simulink model "CF016A_GmVehSpdArbn"  (R2013b)
settings: Solver=FixedStepDiscrete  SolverMode=SingleTasking  StartTime=0.0  StopTime=1  FixedStep=0.002  RelTol=1e-3
undefined symbols (not defined in the file): DIAGCSTRTUPDLY_CNT_U32, NODEBSTEP_CNT_U16, NtcNr1, NtcSts1, VEHSPDMAX_KPH_F32
libraries: simulink x8, NxtrMax x7, NxtrMin x3, NxtrLim x3
(part 2 of 5)

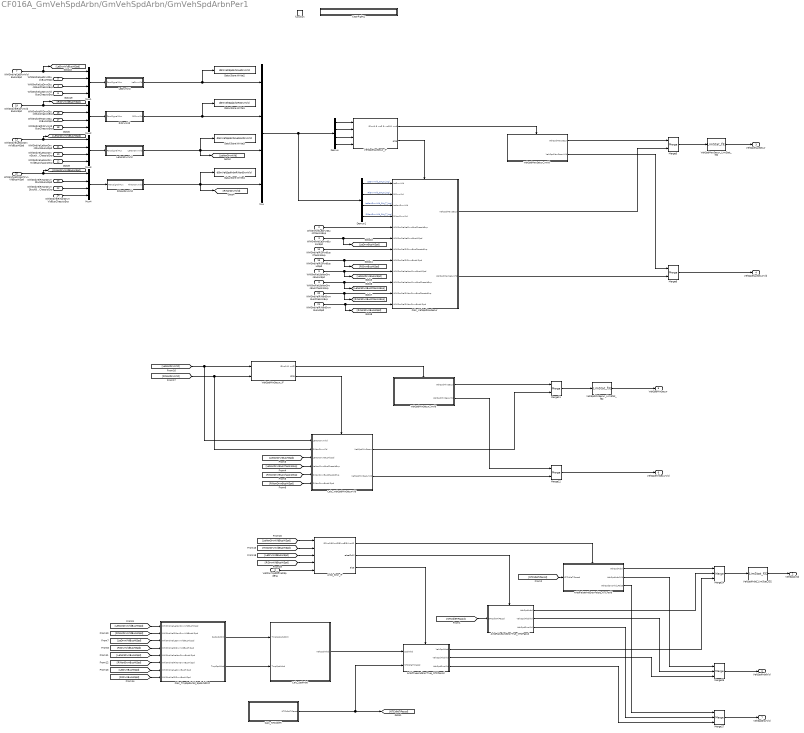
== system CF016A_GmVehSpdArbn/GmVehSpdArbn/GmVehSpdArbnPer1 ==
  VehPwrModDftVehSpdEna : Inport  RequirementInfo="{'linktype_rmi_doors' '0000c6e6 (/GM T1XX/SubSystem Specifications/Customer Functions/CF016A GM Vehicle Speed Arbitration)' '#201' 'true' 'REQ:  201' '' ; 'linktype_rmi_doors' '0000c6e6 (/GM T1XX/SubSystem Specifications/Customer Functions/CF016A GM Vehicle Speed Arbitration)' '#216' 'true' 'REQ:  216' '' ; 'linktype_rmi_doors' '0000c6e6 (/GM T1XX/SubSystem Specifications/Customer Functions/CF016A GM Vehicle Speed Arbitration)' '#55' 'true' 'REQ:  55' '' ; 'linktype_rmi_doors' '0000c6e6 (/GM T1XX/SubSystem Specifications/Customer Functions/CF016A GM Vehicle Speed Arbitration)' '#21' 'true' 'REQ:  21' '' } %GIDa_c4e3bc18_0570_4b3f_a567_ab326b125ca6"  OutDataTypeStr=boolean
  WhlGndVelLeDrvnBusChassisExp : Inport  RequirementInfo="{'linktype_rmi_doors' '0000c6e6 (/GM T1XX/SubSystem Specifications/Customer Functions/CF016A GM Vehicle Speed Arbitration)' '#191' 'true' 'REQ:  191' '' } %GIDa_ef8bad56_b133_4efc_80e4_91ff1fcc71c4"  Port=2
  WhlGndVelLeDrvnBusHiSpd : Inport  RequirementInfo="{'linktype_rmi_doors' '0000c6e6 (/GM T1XX/SubSystem Specifications/Customer Functions/CF016A GM Vehicle Speed Arbitration)' '#191' 'true' 'REQ:  191' '' } %GIDa_139f3ad9_9f11_4eb8_ab0a_dd581ed38c16"  Port=3  OutDataTypeStr=single
  WhlGndVelLeDrvnStuckBusChassisExp : Inport  RequirementInfo="{'linktype_rmi_doors' '0000c6e6 (/GM T1XX/SubSystem Specifications/Customer Functions/CF016A GM Vehicle Speed Arbitration)' '#134' 'true' 'REQ:  134' '' } %GIDa_c2bb7793_67d4_43d9_8d0a_b84d2c7b072b"  Port=4  OutDataTypeStr=boolean
  WhlGndVelLeDrvnStuckBusHiSpd : Inport  RequirementInfo="{'linktype_rmi_doors' '0000c6e6 (/GM T1XX/SubSystem Specifications/Customer Functions/CF016A GM Vehicle Speed Arbitration)' '#134' 'true' 'REQ:  134' '' } %GIDa_c2f775a0_a216_4248_84ff_240bf61a6a65"  Port=5  OutDataTypeStr=boolean
  WhlGndVelLeDrvnVldBusChassisExp : Inport  RequirementInfo="{'linktype_rmi_doors' '0000c6e6 (/GM T1XX/SubSystem Specifications/Customer Functions/CF016A GM Vehicle Speed Arbitration)' '#134' 'true' 'REQ:  134' '' } %GIDa_795613aa_d3d4_4fbe_b3d8_2164d5b0da85"  Port=6  OutDataTypeStr=boolean
  WhlGndVelLeDrvnVldBusHiSpd : Inport  RequirementInfo="{'linktype_rmi_doors' '0000c6e6 (/GM T1XX/SubSystem Specifications/Customer Functions/CF016A GM Vehicle Speed Arbitration)' '#134' 'true' 'REQ:  134' '' } %GIDa_19a58a62_ea8b_42ac_976c_f323a4e5fb4e"  Port=7  OutDataTypeStr=boolean
  WhlGndVelLeNonDrvnBusChassisExp : Inport  RequirementInfo="{'linktype_rmi_doors' '0000c6e6 (/GM T1XX/SubSystem Specifications/Customer Functions/CF016A GM Vehicle Speed Arbitration)' '#191' 'true' 'REQ:  191' '' } %GIDa_816f3292_2a80_407e_aff3_aeaf91f0e3dd"  Port=8  OutDataTypeStr=single
  WhlGndVelLeNonDrvnBusHiSpd : Inport  RequirementInfo="{'linktype_rmi_doors' '0000c6e6 (/GM T1XX/SubSystem Specifications/Customer Functions/CF016A GM Vehicle Speed Arbitration)' '#191' 'true' 'REQ:  191' '' } %GIDa_66072834_5e26_43f6_80a8_02e13e05472d"  Port=9  OutDataTypeStr=single
  WhlGndVelLeNonDrvnStuckBusChassisExp : Inport  RequirementInfo="{'linktype_rmi_doors' '0000c6e6 (/GM T1XX/SubSystem Specifications/Customer Functions/CF016A GM Vehicle Speed Arbitration)' '#164' 'true' 'REQ:  164' '' } %GIDa_721a9ccb_d43e_4602_b1ac_eff13d3c585f"  Port=10  OutDataTypeStr=boolean
  WhlGndVelLeNonDrvnStuckBusHiSpd : Inport  RequirementInfo="{'linktype_rmi_doors' '0000c6e6 (/GM T1XX/SubSystem Specifications/Customer Functions/CF016A GM Vehicle Speed Arbitration)' '#164' 'true' 'REQ:  164' '' } %GIDa_3e912ca7_7856_471d_9266_b6036fbfae10"  Port=11  OutDataTypeStr=boolean
  WhlGndVelLeNonDrvnVldBusChassisExp : Inport  RequirementInfo="{'linktype_rmi_doors' '0000c6e6 (/GM T1XX/SubSystem Specifications/Customer Functions/CF016A GM Vehicle Speed Arbitration)' '#164' 'true' 'REQ:  164' '' } %GIDa_c6bce6c8_b68d_4bb8_bf53_f5356151d1e8"  Port=12  OutDataTypeStr=boolean
  WhlGndVelLeNonDrvnVldBusHiSpd : Inport  RequirementInfo="{'linktype_rmi_doors' '0000c6e6 (/GM T1XX/SubSystem Specifications/Customer Functions/CF016A GM Vehicle Speed Arbitration)' '#164' 'true' 'REQ:  164' '' } %GIDa_c358ba99_35ee_4eda_aec4_59a7f9c2cd81"  Port=13  OutDataTypeStr=boolean
  WhlGndVelRiDrvnBusChassisExp : Inport  RequirementInfo="{'linktype_rmi_doors' '0000c6e6 (/GM T1XX/SubSystem Specifications/Customer Functions/CF016A GM Vehicle Speed Arbitration)' '#191' 'true' 'REQ:  191' '' } %GIDa_5439fa4c_592a_4772_9e24_8e09c86df0d9"  Port=14  OutDataTypeStr=single
  WhlGndVelRiDrvnBusHiSpd : Inport  RequirementInfo="{'linktype_rmi_doors' '0000c6e6 (/GM T1XX/SubSystem Specifications/Customer Functions/CF016A GM Vehicle Speed Arbitration)' '#191' 'true' 'REQ:  191' '' } %GIDa_86c7eb5f_4f31_4eb8_8830_e40c7608a3bf"  Port=15  OutDataTypeStr=single
  WhlGndVelRiDrvnStuckBusChassisExp : Inport  RequirementInfo="{'linktype_rmi_doors' '0000c6e6 (/GM T1XX/SubSystem Specifications/Customer Functions/CF016A GM Vehicle Speed Arbitration)' '#148' 'true' 'REQ:  148' '' } %GIDa_585d7967_0ef8_49d7_8f11_a16ff24051d9"  Port=16  OutDataTypeStr=boolean
  WhlGndVelRiDrvnStuckBusHiSpd : Inport  RequirementInfo="{'linktype_rmi_doors' '0000c6e6 (/GM T1XX/SubSystem Specifications/Customer Functions/CF016A GM Vehicle Speed Arbitration)' '#148' 'true' 'REQ:  148' '' } %GIDa_76749fa7_0454_416a_acff_281ae28f658b"  Port=17  OutDataTypeStr=boolean
  WhlGndVelRiDrvnVldBusChassisExp : Inport  RequirementInfo="{'linktype_rmi_doors' '0000c6e6 (/GM T1XX/SubSystem Specifications/Customer Functions/CF016A GM Vehicle Speed Arbitration)' '#148' 'true' 'REQ:  148' '' } %GIDa_926dc97e_3db9_4017_9435_0a4137e9631c"  Port=18  OutDataTypeStr=boolean
  WhlGndVelRiDrvnVldBusHiSpd : Inport  RequirementInfo="{'linktype_rmi_doors' '0000c6e6 (/GM T1XX/SubSystem Specifications/Customer Functions/CF016A GM Vehicle Speed Arbitration)' '#148' 'true' 'REQ:  148' '' } %GIDa_5fab8672_ee1b_46d3_b7a0_1f2522ac3128"  Port=19  OutDataTypeStr=boolean
  WhlGndVelRiNonDrvnBusChassisExp : Inport  RequirementInfo="{'linktype_rmi_doors' '0000c6e6 (/GM T1XX/SubSystem Specifications/Customer Functions/CF016A GM Vehicle Speed Arbitration)' '#191' 'true' 'REQ:  191' '' } %GIDa_0d94133d_0a6e_49b6_947e_7364e274fe67"  Port=20  OutDataTypeStr=single
  WhlGndVelRiNonDrvnBusHiSpd : Inport  RequirementInfo="{'linktype_rmi_doors' '0000c6e6 (/GM T1XX/SubSystem Specifications/Customer Functions/CF016A GM Vehicle Speed Arbitration)' '#191' 'true' 'REQ:  191' '' } %GIDa_38490758_a269_42a5_8fec_e940c94565d1"  Port=21  OutDataTypeStr=single
  WhlGndVelRiNonDrvnStuckBusChassisExp : Inport  RequirementInfo="{'linktype_rmi_doors' '0000c6e6 (/GM T1XX/SubSystem Specifications/Customer Functions/CF016A GM Vehicle Speed Arbitration)' '#165' 'true' 'REQ:  165' '' } %GIDa_e0cb1563_d840_4dd2_a90a_2d810a7a7354"  Port=22  OutDataTypeStr=boolean
  WhlGndVelRiNonDrvnStuckBusHiSpd : Inport  RequirementInfo="{'linktype_rmi_doors' '0000c6e6 (/GM T1XX/SubSystem Specifications/Customer Functions/CF016A GM Vehicle Speed Arbitration)' '#165' 'true' 'REQ:  165' '' } %GIDa_e31240b4_81cc_4ab0_98ca_8ec14bb44c74"  Port=23  OutDataTypeStr=boolean
  WhlGndVelRiNonDrvnVldBusChassisExp : Inport  RequirementInfo="{'linktype_rmi_doors' '0000c6e6 (/GM T1XX/SubSystem Specifications/Customer Functions/CF016A GM Vehicle Speed Arbitration)' '#165' 'true' 'REQ:  165' '' } %GIDa_7a5865c5_6788_4082_bc3e_71db9840dce9"  Port=24  OutDataTypeStr=boolean
  WhlGndVelRiNonDrvnVldBusHiSpd : Inport  RequirementInfo="{'linktype_rmi_doors' '0000c6e6 (/GM T1XX/SubSystem Specifications/Customer Functions/CF016A GM Vehicle Speed Arbitration)' '#165' 'true' 'REQ:  165' '' } %GIDa_97efc4a3_badf_4f9c_a1b1_7d9397b8ff86"  Port=25  OutDataTypeStr=boolean
  function : TriggerPort  TriggerType=function-call
  ArbdFalseAndSnsrFalse_NTCFaild : Subsystem  RequirementInfo="{'linktype_rmi_doors' '0000c6e6 (/GM T1XX/SubSystem Specifications/Customer Functions/CF016A GM Vehicle Speed Arbitration)' '#201' 'true' 'REQ:  201' '' ; 'linktype_rmi_doors' '0000c6e6 (/GM T1XX/SubSystem Specifications/Customer Functions/CF016A GM Vehicle Speed Arbitration)' '#216' 'true' 'REQ:  216' '' ; 'linktype_rmi_doors' '0000c6e6 (/GM T1XX/SubSystem Specifications/Customer Functions/CF016A GM Vehicle Speed Arbitration)' '#55' 'true' 'REQ:  55' '' } %GIDa_a2946cc7_76d5_475e_a7d4_3e59e6c0f436"  TreatAsAtomicUnit=on
  ArbdFalseAndSnsrTrue_NTCPassd : Subsystem  RequirementInfo="{'linktype_rmi_doors' '0000c6e6 (/GM T1XX/SubSystem Specifications/Customer Functions/CF016A GM Vehicle Speed Arbitration)' '#201' 'true' 'REQ:  201' '' ; 'linktype_rmi_doors' '0000c6e6 (/GM T1XX/SubSystem Specifications/Customer Functions/CF016A GM Vehicle Speed Arbitration)' '#216' 'true' 'REQ:  216' '' ; 'linktype_rmi_doors' '0000c6e6 (/GM T1XX/SubSystem Specifications/Customer Functions/CF016A GM Vehicle Speed Arbitration)' '#55' 'true' 'REQ:  55' '' ; 'linktype_rmi_doors' '0000c6e6 (/GM T1XX/SubSystem Specifications/Customer Functions/CF016A GM Vehicle Speed Arbitration)' '#21' 'true' 'REQ:  21' '' } %GIDa_24968ccd_650a_4f02_a76c_60fb17be485c"  TreatAsAtomicUnit=on
  ArbdTrueAndSnsrTrue_NTCPassd : Subsystem  RequirementInfo="{'linktype_rmi_doors' '0000c6e6 (/GM T1XX/SubSystem Specifications/Customer Functions/CF016A GM Vehicle Speed Arbitration)' '#201' 'true' 'REQ:  201' '' ; 'linktype_rmi_doors' '0000c6e6 (/GM T1XX/SubSystem Specifications/Customer Functions/CF016A GM Vehicle Speed Arbitration)' '#216' 'true' 'REQ:  216' '' ; 'linktype_rmi_doors' '0000c6e6 (/GM T1XX/SubSystem Specifications/Customer Functions/CF016A GM Vehicle Speed Arbitration)' '#55' 'true' 'REQ:  55' '' } %GIDa_a93f8941_36e9_423e_8493_7bbaddef002d"  TreatAsAtomicUnit=on
  Arbd_Snsr_IF : If  RequirementInfo="{'linktype_rmi_doors' '0000c6e6 (/GM T1XX/SubSystem Specifications/Customer Functions/CF016A GM Vehicle Speed Arbitration)' '#201' 'true' 'REQ:  201' '' ; 'linktype_rmi_doors' '0000c6e6 (/GM T1XX/SubSystem Specifications/Customer Functions/CF016A GM Vehicle Speed Arbitration)' '#216' 'true' 'REQ:  216' '' ; 'linktype_rmi_doors' '0000c6e6 (/GM T1XX/SubSystem Specifications/Customer Functions/CF016A GM Vehicle Speed Arbitration)' '#55' 'true' 'REQ:  55' '' ; 'linktype_rmi_doors' '0000c6e6 (/GM T1XX/SubSystem Specifications/Customer Functions/CF016A GM Vehicle Speed Arbitration)' '#21' 'true' 'REQ:  21' '' } %GIDa_cd7d7c1a_47a2_4b6f_81bf_446ff4509ba4"  NumInputs=5  IfExpression=(~u1)&(~u2)&(~u3)&(~u4)  ElseIfExpressions=u5
      settings: AttributesFormatString=|
      | IF: %<IfExpression>
      | ELSE IF: %<ElseIfExpressions>
  Calc_NTCIdleTi : Subsystem  RequirementInfo="{'linktype_rmi_doors' '0000c6e6 (/GM T1XX/SubSystem Specifications/Customer Functions/CF016A GM Vehicle Speed Arbitration)' '#223' 'true' 'REQ:  223' '' } %GIDa_b1c70a04_ae11_4796_80c0_e305c1af5713"
  Calc_SpdArbd : Subsystem  RequirementInfo="{'linktype_rmi_doors' '0000c6e6 (/GM T1XX/SubSystem Specifications/Customer Functions/CF016A GM Vehicle Speed Arbitration)' '#197' 'true' 'REQ:  197' '' } %GIDa_16311984_c18c_4fe4_ad8c_ca1138d95f11"
  Calc_TmpSpdArbd_SpdArbdCnt : Subsystem  RequirementInfo="{'linktype_rmi_doors' '0000c6e6 (/GM T1XX/SubSystem Specifications/Customer Functions/CF016A GM Vehicle Speed Arbitration)' '#197' 'true' 'REQ:  197' '' } %GIDa_bc6bf8a9_5351_4ff1_8876_c778375d82ed"
  Calc_VehSpdMaxSecur : Subsystem  RequirementInfo="{'linktype_rmi_doors' '0000c6e6 (/GM T1XX/SubSystem Specifications/Customer Functions/CF016A GM Vehicle Speed Arbitration)' '#42' 'true' 'REQ:  42' '' } %GIDa_18b5dd71_8b65_4e5b_b3d7_592b4660d087"  TreatAsAtomicUnit=on
  Calc_VehSpdMinSecurVld : Subsystem  RequirementInfo="{'linktype_rmi_doors' '0000c6e6 (/GM T1XX/SubSystem Specifications/Customer Functions/CF016A GM Vehicle Speed Arbitration)' '#200' 'true' 'REQ:  200' '' } %GIDa_87f42618_bdcc_4508_97d2_5a3f6cb92617"  TreatAsAtomicUnit=on
  CopyRight2 : Subsystem  Description=|  mask(Copyright Information){none=on}
      | Copyright info block.                                               
      |                                                                     
      | Place copyright information at the top of every subsystem in design.
      mask prompts: none "No parameters"
      mask help: Place copyright information at the top of every subsystem in design.
      mask Display:
      | NxtrConf = 'Nexteer Confidential';
      | 
      | sys = bdroot; %handle for the current model ("system")
      | first = get_param(sys,'Created');
      | if(isempty(first))
      |     first = datestr(now,'yyyy');
      | else
      |     first = first(end-3:end);  %year is last four digits
      | end
      | 
      | last = get_param(sys,'LastModifiedDate');
      | if isempty(last)
      |     last = datestr(now,'yyyy');
      | else
      |     last = last(end-3:end);
      | end
      | 
      | if strcmp(first,last)
      |     fprintf('%s -- Copyright %s Nexteer',NxtrConf,first)
      | else
      |     fprintf('%s -- %s%s- %s Nexteer',NxtrConf,char(169),first,last)
      | end
  Data Store Write1 : DataStoreWrite  RequirementInfo="{'linktype_rmi_doors' '0000c6e6 (/GM T1XX/SubSystem Specifications/Customer Functions/CF016A GM Vehicle Speed Arbitration)' '#148' 'true' 'REQ:  148' '' } %GIDa_65a22cee_f7c3_4e4f_9841_3f731132c91b"  DataStoreName=dGmVehSpdArbnRiDrvnVld
  Data Store Write2 : DataStoreWrite  RequirementInfo="{'linktype_rmi_doors' '0000c6e6 (/GM T1XX/SubSystem Specifications/Customer Functions/CF016A GM Vehicle Speed Arbitration)' '#134' 'true' 'REQ:  134' '' } %GIDa_6506a920_d21b_4a41_8912_67910f5698ca"  DataStoreName=dGmVehSpdArbnLeDrvnVld
  Data Store Write3 : DataStoreWrite  RequirementInfo="{'linktype_rmi_doors' '0000c6e6 (/GM T1XX/SubSystem Specifications/Customer Functions/CF016A GM Vehicle Speed Arbitration)' '#164' 'true' 'REQ:  164' '' } %GIDa_7caea8aa_01ba_480f_a0e3_d7874300fc26"  DataStoreName=dGmVehSpdArbnLeNonDrvnVld
  Data Store Write4 : DataStoreWrite  RequirementInfo="{'linktype_rmi_doors' '0000c6e6 (/GM T1XX/SubSystem Specifications/Customer Functions/CF016A GM Vehicle Speed Arbitration)' '#165' 'true' 'REQ:  165' '' } %GIDa_537405e5_2b08_46e6_bc5f_2c920737d5d3"  DataStoreName=dGmVehSpdArbnRiNonDrvnVld
  Demux : Demux  RequirementInfo="{'linktype_rmi_doors' '0000c6e6 (/GM T1XX/SubSystem Specifications/Customer Functions/CF016A GM Vehicle Speed Arbitration)' '#151' 'true' 'REQ:  151' '' } %GIDa_9996e851_1594_4344_ab35_741cd3cb2f5f"
  Demux1 : Demux
  LeDrvnVld : Subsystem  RequirementInfo="{'linktype_rmi_doors' '0000c6e6 (/GM T1XX/SubSystem Specifications/Customer Functions/CF016A GM Vehicle Speed Arbitration)' '#134' 'true' 'REQ:  134' '' } %GIDa_91d91c9c_e4ce_47bd_8edb_064a3de60f07"
  LeNonDrvnVld : Subsystem  RequirementInfo="{'linktype_rmi_doors' '0000c6e6 (/GM T1XX/SubSystem Specifications/Customer Functions/CF016A GM Vehicle Speed Arbitration)' '#164' 'true' 'REQ:  164' '' } %GIDa_738d4c5d_c85c_4fc7_a21b_b06397be08db"
  Merge11 : Merge  RequirementInfo="{'linktype_rmi_doors' '0000c6e6 (/GM T1XX/SubSystem Specifications/Customer Functions/CF016A GM Vehicle Speed Arbitration)' '#200' 'true' 'REQ:  200' '' } %GIDa_c6f44c10_058a_4ce8_bab9_d9e154170ef5"
  Merge12 : Merge  RequirementInfo="{'linktype_rmi_doors' '0000c6e6 (/GM T1XX/SubSystem Specifications/Customer Functions/CF016A GM Vehicle Speed Arbitration)' '#200' 'true' 'REQ:  200' '' } %GIDa_5ca221ae_a0a0_4349_801e_90a121427c6f"
  Merge24 : Merge  RequirementInfo="{'linktype_rmi_doors' '0000c6e6 (/GM T1XX/SubSystem Specifications/Customer Functions/CF016A GM Vehicle Speed Arbitration)' '#201' 'true' 'REQ:  201' '' ; 'linktype_rmi_doors' '0000c6e6 (/GM T1XX/SubSystem Specifications/Customer Functions/CF016A GM Vehicle Speed Arbitration)' '#216' 'true' 'REQ:  216' '' ; 'linktype_rmi_doors' '0000c6e6 (/GM T1XX/SubSystem Specifications/Customer Functions/CF016A GM Vehicle Speed Arbitration)' '#55' 'true' 'REQ:  55' '' } %GIDa_74dbaf74_bffd_42bd_8f7c_be8132b0f70d"  Inputs=3
  Merge25 : Merge  RequirementInfo="{'linktype_rmi_doors' '0000c6e6 (/GM T1XX/SubSystem Specifications/Customer Functions/CF016A GM Vehicle Speed Arbitration)' '#201' 'true' 'REQ:  201' '' ; 'linktype_rmi_doors' '0000c6e6 (/GM T1XX/SubSystem Specifications/Customer Functions/CF016A GM Vehicle Speed Arbitration)' '#216' 'true' 'REQ:  216' '' ; 'linktype_rmi_doors' '0000c6e6 (/GM T1XX/SubSystem Specifications/Customer Functions/CF016A GM Vehicle Speed Arbitration)' '#55' 'true' 'REQ:  55' '' } %GIDa_f96da6f3_b28c_497a_a08f_fa4ee1d04650"  Inputs=3
  Merge27 : Merge  RequirementInfo="{'linktype_rmi_doors' '0000c6e6 (/GM T1XX/SubSystem Specifications/Customer Functions/CF016A GM Vehicle Speed Arbitration)' '#201' 'true' 'REQ:  201' '' ; 'linktype_rmi_doors' '0000c6e6 (/GM T1XX/SubSystem Specifications/Customer Functions/CF016A GM Vehicle Speed Arbitration)' '#216' 'true' 'REQ:  216' '' ; 'linktype_rmi_doors' '0000c6e6 (/GM T1XX/SubSystem Specifications/Customer Functions/CF016A GM Vehicle Speed Arbitration)' '#55' 'true' 'REQ:  55' '' } %GIDa_6c6a62b5_c7c1_4c08_997c_c80f62d1f379"  Inputs=3
  Merge5 : Merge  RequirementInfo="{'linktype_rmi_doors' '0000c6e6 (/GM T1XX/SubSystem Specifications/Customer Functions/CF016A GM Vehicle Speed Arbitration)' '#151' 'true' 'REQ:  151' '' } %GIDa_acbd5b31_4090_4db2_ab19_fa88f3c82fb7"
  Merge6 : Merge  RequirementInfo="{'linktype_rmi_doors' '0000c6e6 (/GM T1XX/SubSystem Specifications/Customer Functions/CF016A GM Vehicle Speed Arbitration)' '#112' 'true' 'REQ:  112' '' } %GIDa_ca72796b_2adb_4b6b_a64e_123863fd010f"
  Mux : Mux
  Mux1 : Mux  RequirementInfo="{'linktype_rmi_doors' '0000c6e6 (/GM T1XX/SubSystem Specifications/Customer Functions/CF016A GM Vehicle Speed Arbitration)' '#134' 'true' 'REQ:  134' '' } %GIDa_8538414b_2453_4e81_a0f3_b9ebfcd930a3"
  Mux2 : Mux  RequirementInfo="{'linktype_rmi_doors' '0000c6e6 (/GM T1XX/SubSystem Specifications/Customer Functions/CF016A GM Vehicle Speed Arbitration)' '#148' 'true' 'REQ:  148' '' } %GIDa_33455157_8d31_4396_ae6e_87ab98132e28"
  Mux3 : Mux  RequirementInfo="{'linktype_rmi_doors' '0000c6e6 (/GM T1XX/SubSystem Specifications/Customer Functions/CF016A GM Vehicle Speed Arbitration)' '#164' 'true' 'REQ:  164' '' } %GIDa_6ff3f051_e4fb_48ea_90e3_2c2101f1141a"
  Mux4 : Mux  RequirementInfo="{'linktype_rmi_doors' '0000c6e6 (/GM T1XX/SubSystem Specifications/Customer Functions/CF016A GM Vehicle Speed Arbitration)' '#165' 'true' 'REQ:  165' '' } %GIDa_29a8bb81_be2d_4f2f_8ddf_846dcde25de1"
  RiDrvnVld : Subsystem  RequirementInfo="{'linktype_rmi_doors' '0000c6e6 (/GM T1XX/SubSystem Specifications/Customer Functions/CF016A GM Vehicle Speed Arbitration)' '#148' 'true' 'REQ:  148' '' } %GIDa_a811e6bb_3949_43cf_9154_0874718e5d03"
  RiNonDrvnVld : Subsystem  RequirementInfo="{'linktype_rmi_doors' '0000c6e6 (/GM T1XX/SubSystem Specifications/Customer Functions/CF016A GM Vehicle Speed Arbitration)' '#165' 'true' 'REQ:  165' '' } %GIDa_70fe0848_1c8f_420c_80b5_ca04f38782e1"
  VehSpdArbd_LimStat_f32 : NxtrLim/LimStat_f32  RequirementInfo="{'linktype_rmi_doors' '0000c6e6 (/GM T1XX/SubSystem Specifications/Customer Functions/CF016A GM Vehicle Speed Arbitration)' '#201' 'true' 'REQ:  201' '' ; 'linktype_rmi_doors' '0000c6e6 (/GM T1XX/SubSystem Specifications/Customer Functions/CF016A GM Vehicle Speed Arbitration)' '#216' 'true' 'REQ:  216' '' ; 'linktype_rmi_doors' '0000c6e6 (/GM T1XX/SubSystem Specifications/Customer Functions/CF016A GM Vehicle Speed Arbitration)' '#55' 'true' 'REQ:  55' '' } %GIDa_7623a915_6304_4bff_9a32_a22773e0171a"  LoLim=VEHSPDMIN_KPH_F32  HiLim=VEHSPDMAX_KPH_F32
      settings: AttributesFormatString=|
      | Low Limit: %<LoLim>
      | High Limit:%<HiLim>
  VehSpdMaxSecur_IF : If  RequirementInfo="{'linktype_rmi_doors' '0000c6e6 (/GM T1XX/SubSystem Specifications/Customer Functions/CF016A GM Vehicle Speed Arbitration)' '#151' 'true' 'REQ:  151' '' } %GIDa_255fb6b3_53ca_44c6_bfbf_9117d93cbb61"  NumInputs=4  IfExpression=~u1 & ~u2 & ~u3 & ~u4
      settings: AttributesFormatString=IF: %<IfExpression>
  VehSpdMaxSecur_Invld : Subsystem  RequirementInfo="{'linktype_rmi_doors' '0000c6e6 (/GM T1XX/SubSystem Specifications/Customer Functions/CF016A GM Vehicle Speed Arbitration)' '#151' 'true' 'REQ:  151' '' } %GIDa_26113a26_743f_47ad_b9d5_0957c18d60fe"  TreatAsAtomicUnit=on
  VehSpdMaxSecur_LimStat_f32 : NxtrLim/LimStat_f32  RequirementInfo="{'linktype_rmi_doors' '0000c6e6 (/GM T1XX/SubSystem Specifications/Customer Functions/CF016A GM Vehicle Speed Arbitration)' '#151' 'true' 'REQ:  151' '' } %GIDa_5098e77a_229a_4468_9465_403b3d7a857f"  LoLim=VEHSPDMIN_KPH_F32  HiLim=VEHSPDMAX_KPH_F32
      settings: AttributesFormatString=|
      | Low Limit: %<LoLim>
      | High Limit:%<HiLim>
  VehSpdMinSecur_IF : If  RequirementInfo="{'linktype_rmi_doors' '0000c6e6 (/GM T1XX/SubSystem Specifications/Customer Functions/CF016A GM Vehicle Speed Arbitration)' '#200' 'true' 'REQ:  200' '' } %GIDa_25ca72f0_ada2_41b1_aa48_2ee7a36aa6a8"  NumInputs=2  IfExpression=~u1 & ~u2
      settings: AttributesFormatString=%<Priority>
  VehSpdMinSecur_Invld : Subsystem  RequirementInfo="{'linktype_rmi_doors' '0000c6e6 (/GM T1XX/SubSystem Specifications/Customer Functions/CF016A GM Vehicle Speed Arbitration)' '#200' 'true' 'REQ:  200' '' } %GIDa_23e9f4eb_eb52_4411_b903_b362a0e45c28"  TreatAsAtomicUnit=on
  VehSpdMinSecur_LimStat_f32 : NxtrLim/LimStat_f32  RequirementInfo="{'linktype_rmi_doors' '0000c6e6 (/GM T1XX/SubSystem Specifications/Customer Functions/CF016A GM Vehicle Speed Arbitration)' '#200' 'true' 'REQ:  200' '' } %GIDa_81eb093f_12a4_4da7_990c_8a1096a9d65e"  LoLim=VEHSPDMIN_KPH_F32  HiLim=VEHSPDMAX_KPH_F32
      settings: AttributesFormatString=|
      | Low Limit: %<LoLim>
      | High Limit:%<HiLim>
  VehSpdArbd : Outport  RequirementInfo="{'linktype_rmi_doors' '0000c6e6 (/GM T1XX/SubSystem Specifications/Customer Functions/CF016A GM Vehicle Speed Arbitration)' '#201' 'true' 'REQ:  201' '' ; 'linktype_rmi_doors' '0000c6e6 (/GM T1XX/SubSystem Specifications/Customer Functions/CF016A GM Vehicle Speed Arbitration)' '#216' 'true' 'REQ:  216' '' ; 'linktype_rmi_doors' '0000c6e6 (/GM T1XX/SubSystem Specifications/Customer Functions/CF016A GM Vehicle Speed Arbitration)' '#55' 'true' 'REQ:  55' '' } %GIDa_3e9161e8_922c_4bad_9ff1_99368e418145"
  VehSpdArbdVld : Outport  RequirementInfo="{'linktype_rmi_doors' '0000c6e6 (/GM T1XX/SubSystem Specifications/Customer Functions/CF016A GM Vehicle Speed Arbitration)' '#201' 'true' 'REQ:  201' '' ; 'linktype_rmi_doors' '0000c6e6 (/GM T1XX/SubSystem Specifications/Customer Functions/CF016A GM Vehicle Speed Arbitration)' '#216' 'true' 'REQ:  216' '' ; 'linktype_rmi_doors' '0000c6e6 (/GM T1XX/SubSystem Specifications/Customer Functions/CF016A GM Vehicle Speed Arbitration)' '#55' 'true' 'REQ:  55' '' } %GIDa_09f612c1_4377_4556_992f_978cffce312c"  Port=2
  VehSpdMaxSecur : Outport  RequirementInfo="{'linktype_rmi_doors' '0000c6e6 (/GM T1XX/SubSystem Specifications/Customer Functions/CF016A GM Vehicle Speed Arbitration)' '#151' 'true' 'REQ:  151' '' } %GIDa_5131550b_ffe5_4928_911d_89cceeef0f6f"  Port=3
  VehSpdMaxSecurVld : Outport  RequirementInfo="{'linktype_rmi_doors' '0000c6e6 (/GM T1XX/SubSystem Specifications/Customer Functions/CF016A GM Vehicle Speed Arbitration)' '#112' 'true' 'REQ:  112' '' } %GIDa_d4b7e114_9196_4ce1_ab50_3a87cb5bfc07"  Port=4
  VehSpdMinSecur : Outport  RequirementInfo="{'linktype_rmi_doors' '0000c6e6 (/GM T1XX/SubSystem Specifications/Customer Functions/CF016A GM Vehicle Speed Arbitration)' '#200' 'true' 'REQ:  200' '' } %GIDa_a06c0167_4d35_4ddd_bc02_fac87e130614"  Port=5
  VehSpdMinSecurVld : Outport  RequirementInfo="{'linktype_rmi_doors' '0000c6e6 (/GM T1XX/SubSystem Specifications/Customer Functions/CF016A GM Vehicle Speed Arbitration)' '#200' 'true' 'REQ:  200' '' } %GIDa_192cc651_13b8_49be_9832_0fd36d1db41b"  Port=6
  VehSpdSnsrVld : Outport  RequirementInfo="{'linktype_rmi_doors' '0000c6e6 (/GM T1XX/SubSystem Specifications/Customer Functions/CF016A GM Vehicle Speed Arbitration)' '#201' 'true' 'REQ:  201' '' ; 'linktype_rmi_doors' '0000c6e6 (/GM T1XX/SubSystem Specifications/Customer Functions/CF016A GM Vehicle Speed Arbitration)' '#216' 'true' 'REQ:  216' '' ; 'linktype_rmi_doors' '0000c6e6 (/GM T1XX/SubSystem Specifications/Customer Functions/CF016A GM Vehicle Speed Arbitration)' '#55' 'true' 'REQ:  55' '' } %GIDa_cb101305_07ae_4f10_b1b4_ec7d7ab6413d"  Port=7
  wires:
  VehSpdMaxSecur_IF/1 -> VehSpdMaxSecur_Invld/Action
  VehSpdMaxSecur_IF/2 -> Calc_VehSpdMaxSecur/Action
  VehSpdMaxSecur_Invld/1(VehSpdMaxSecur) -> Merge5/1
  Calc_VehSpdMaxSecur/1(VehSpdMaxSecur) -> Merge5/2
  VehSpdMaxSecur_Invld/2(VehSpdMaxSecurVld) -> Merge6/1
  Calc_VehSpdMaxSecur/2(VehSpdMaxSecurVld) -> Merge6/2
  Merge5/1 -> VehSpdMaxSecur_LimStat_f32/1
  Merge6/1 -> VehSpdMaxSecurVld/1
  [LeNonDrvnVld] -> Calc_VehSpdMinSecurVld/1(LeNonDrvnVld), VehSpdMinSecur_IF/1
  [RiNonDrvnVld] -> Calc_VehSpdMinSecurVld/2(RiNonDrvnVld), VehSpdMinSecur_IF/2
  VehSpdMinSecur_IF/1 -> VehSpdMinSecur_Invld/Action
  VehSpdMinSecur_IF/2 -> Calc_VehSpdMinSecurVld/Action
  VehSpdMinSecur_Invld/1(VehSpdMinSecur) -> Merge11/1
  Calc_VehSpdMinSecurVld/1(VehSpdMinSecur) -> Merge11/2
  VehSpdMinSecur_Invld/2(VehSpdMinSecurVld) -> Merge12/1
  Calc_VehSpdMinSecurVld/2(VehSpdMinSecurVld) -> Merge12/2
  Merge11/1 -> VehSpdMinSecur_LimStat_f32/1
  Merge12/1 -> VehSpdMinSecurVld/1
  [LeNonDrvnVldBusHiSpd] -> Arbd_Snsr_IF/1
  [RiNonDrvnVldBusHiSpd] -> Arbd_Snsr_IF/2
  [LeDrvnVldBusHiSpd] -> Arbd_Snsr_IF/3
  [RiDrvnVldBusHiSpd] -> Arbd_Snsr_IF/4
  VehPwrModDftVehSpdEna/1 -> Arbd_Snsr_IF/5
  Arbd_Snsr_IF/1 -> ArbdFalseAndSnsrFalse_NTCFaild/Action
  Arbd_Snsr_IF/3 -> ArbdTrueAndSnsrTrue_NTCPassd/Action
  Merge25/1 -> VehSpdArbdVld/1
  Merge24/1 -> VehSpdArbd_LimStat_f32/1
  Arbd_Snsr_IF/2 -> ArbdFalseAndSnsrTrue_NTCPassd/Action
  [NTCIdleTiPassd] -> ArbdFalseAndSnsrTrue_NTCPassd/1(NTCIdleTiPassd)
  [NTCIdleTiPassd] -> ArbdFalseAndSnsrFalse_NTCFaild/1(NTCIdleTiPassd)
  ArbdFalseAndSnsrFalse_NTCFaild/1(VehSpdArbd) -> Merge24/1
  ArbdFalseAndSnsrTrue_NTCPassd/1(VehSpdArbd) -> Merge24/2
  ArbdTrueAndSnsrTrue_NTCPassd/1(VehSpdArbd) -> Merge24/3
  ArbdFalseAndSnsrFalse_NTCFaild/2(VehSpdArbdVld) -> Merge25/1
  ArbdFalseAndSnsrTrue_NTCPassd/2(VehSpdArbdVld) -> Merge25/2
  ArbdTrueAndSnsrTrue_NTCPassd/2(VehSpdArbdVld) -> Merge25/3
  Merge27/1 -> VehSpdSnsrVld/1
  ArbdFalseAndSnsrFalse_NTCFaild/3(VehSpdSnsrVld_False) -> Merge27/1
  ArbdFalseAndSnsrTrue_NTCPassd/3(VehSpdSnsrVld) -> Merge27/2
  ArbdTrueAndSnsrTrue_NTCPassd/3(VehSpdSnsrVld) -> Merge27/3
  VehSpdMaxSecur_LimStat_f32/1 -> VehSpdMaxSecur/1
  VehSpdMinSecur_LimStat_f32/1 -> VehSpdMinSecur/1
  VehSpdArbd_LimStat_f32/1 -> VehSpdArbd/1
  WhlGndVelLeDrvnBusChassisExp/1 -> Calc_VehSpdMaxSecur/5(WhlGndVelLeDrvnBusChassisExp)
  WhlGndVelRiDrvnBusChassisExp/1 -> Calc_VehSpdMaxSecur/7(WhlGndVelRiDrvnBusChassisExp)
  WhlGndVelRiDrvnBusHiSpd/1 -> [RiDrvnBusHiSpd], Calc_VehSpdMaxSecur/8(WhlGndVelRiDrvnBusHiSpd)
  WhlGndVelLeNonDrvnBusHiSpd/1 -> [LeNonDrvnBusHiSpd], Calc_VehSpdMaxSecur/9(WhlGndVelLeNonDrvnBusHiSpd)
  WhlGndVelLeNonDrvnBusChassisExp/1 -> [LeNonDrvnBusChassisExp], Calc_VehSpdMaxSecur/10(WhlGndVelLeNonDrvnBusChassisExp)
  WhlGndVelRiNonDrvnBusChassisExp/1 -> [RiNonDrvnBusChassisExp], Calc_VehSpdMaxSecur/11(WhlGndVelRiNonDrvnBusChassisExp)
  WhlGndVelRiNonDrvnBusHiSpd/1 -> [RiNonDrvnBusHiSpd], Calc_VehSpdMaxSecur/12(WhlGndVelRiNonDrvnBusHiSpd)
  [LeNonDrvnBusHiSpd] -> Calc_VehSpdMinSecurVld/3(LeNonDrvnBusHiSpd)
  [LeNonDrvnBusChassisExp] -> Calc_VehSpdMinSecurVld/4(LeNonDrvnBusChassisExp)
  [RiNonDrvnBusChassisExp] -> Calc_VehSpdMinSecurVld/5(RiNonDrvnBusChassisExp)
  [RiNonDrvnBusHiSpd] -> Calc_VehSpdMinSecurVld/6(RiNonDrvnBusHiSpd)
  Demux/1 -> VehSpdMaxSecur_IF/1
  Demux/2 -> VehSpdMaxSecur_IF/2
  Demux/3 -> VehSpdMaxSecur_IF/3
  Demux/4 -> VehSpdMaxSecur_IF/4
  Mux/1 -> Demux/1, Demux1/1
  Demux1/2 -> Calc_VehSpdMaxSecur/2(RiDrvnVld)  "RiDrvnVld_Cnt_T_logl"
  Demux1/3 -> Calc_VehSpdMaxSecur/3(LeNonDrvnVld)  "LeNonDrvnVld_Cnt_T_logl"
  Demux1/4 -> Calc_VehSpdMaxSecur/4(RiNonDrvnVld)  "RiNonDrvnVld_Cnt_T_logl"
  WhlGndVelLeDrvnVldBusHiSpd/1 -> [LeDrvnVldBusHiSpd], Mux1/1
  WhlGndVelLeDrvnStuckBusHiSpd/1 -> Mux1/2
  WhlGndVelLeDrvnStuckBusChassisExp/1 -> Mux1/3
  WhlGndVelLeDrvnVldBusChassisExp/1 -> Mux1/4
  Mux1/1 -> LeDrvnVld/1(RawSignalMux)
  WhlGndVelRiDrvnVldBusHiSpd/1 -> [RiDrvnVldBusHiSpd], Mux2/1
  WhlGndVelRiDrvnStuckBusChassisExp/1 -> Mux2/2
  WhlGndVelRiDrvnStuckBusHiSpd/1 -> Mux2/3
  WhlGndVelRiDrvnVldBusChassisExp/1 -> Mux2/4
  Mux2/1 -> RiDrvnVld/1(RawSignalMux)
  WhlGndVelLeNonDrvnStuckBusHiSpd/1 -> Mux3/2
  Mux3/1 -> LeNonDrvnVld/1(RawSignalMux)
  WhlGndVelRiNonDrvnVldBusHiSpd/1 -> Mux4/1, [RiNonDrvnVldBusHiSpd]
  WhlGndVelRiNonDrvnStuckBusHiSpd/1 -> Mux4/2
  WhlGndVelRiNonDrvnStuckBusChassisExp/1 -> Mux4/3
  WhlGndVelRiNonDrvnVldBusChassisExp/1 -> Mux4/4
  Mux4/1 -> RiNonDrvnVld/1(RawSignalMux)
  WhlGndVelLeNonDrvnStuckBusChassisExp/1 -> Mux3/3
  WhlGndVelLeNonDrvnVldBusChassisExp/1 -> Mux3/4
  WhlGndVelLeNonDrvnVldBusHiSpd/1 -> [LeNonDrvnVldBusHiSpd], Mux3/1
  Calc_TmpSpdArbd_SpdArbdCnt/1(SpdArbdCnt) -> Calc_SpdArbd/1(TmpSpdArbdCnt)
  Calc_TmpSpdArbd_SpdArbdCnt/2(TmpSpdArbd) -> Calc_SpdArbd/2(TmpSpdArbd)
  [LeNonDrvnVldBusHiSpd] -> Calc_TmpSpdArbd_SpdArbdCnt/1(WhlGndVelLeNonDrvnVldBusHiSpd)
  [RiNonDrvnVldBusHiSpd] -> Calc_TmpSpdArbd_SpdArbdCnt/2(WhlGndVelRiNonDrvnVldBusHiSpd)
  [LeDrvnVldBusHiSpd] -> Calc_TmpSpdArbd_SpdArbdCnt/3(WhlGndVelLeDrvnVldBusHiSpd)
  [RiDrvnVldBusHiSpd] -> Calc_TmpSpdArbd_SpdArbdCnt/4(WhlGndVelRiDrvnVldBusHiSpd)
  [LeNonDrvnBusHiSpd] -> Calc_TmpSpdArbd_SpdArbdCnt/5(WhlGndVelLeNonDrvnBusHiSpd)
  [RiNonDrvnBusHiSpd] -> Calc_TmpSpdArbd_SpdArbdCnt/6(WhlGndVelRiNonDrvnBusHiSpd)
  WhlGndVelLeDrvnBusHiSpd/1 -> [LeDrvnBusHiSpd], Calc_VehSpdMaxSecur/6(WhlGndVelLeDrvnBusHiSpd)
  [LeDrvnBusHiSpd] -> Calc_TmpSpdArbd_SpdArbdCnt/7(WhlGndVelLeDrvnBusHiSpd)
  [RiDrvnBusHiSpd] -> Calc_TmpSpdArbd_SpdArbdCnt/8(WhlGndVelRiDrvnBusHiSpd)
  Calc_SpdArbd/1(VehSpdArbd) -> ArbdTrueAndSnsrTrue_NTCPassd/1(SpdArbd)
  Calc_NTCIdleTi/1(NTCIdleTiPassd) -> [NTCIdleTiPassd], ArbdTrueAndSnsrTrue_NTCPassd/2(NTCIdleTiPassd)
  LeDrvnVld/1(LeDrvnVld) -> Data Store Write2/1, Mux/1
  RiDrvnVld/1(RiDrvnVld) -> Data Store Write1/1, Mux/2
  LeNonDrvnVld/1(LeNonDrvnVld) -> Data Store Write3/1, [LeNonDrvnVld], Mux/3
  RiNonDrvnVld/1(RiNonDrvnVld) -> Data Store Write4/1, [RiNonDrvnVld], Mux/4
  Demux1/1 -> Calc_VehSpdMaxSecur/1(LeDrvnVld)  "LeDrvnVld_Cnt_T_logl"

== system CF016A_GmVehSpdArbn/call_GmVehSpdArbnInit1/CopyRight2 ==

== system CF016A_GmVehSpdArbn/GmVehSpdArbn/GmVehSpdArbnInit1/CopyRight2 ==

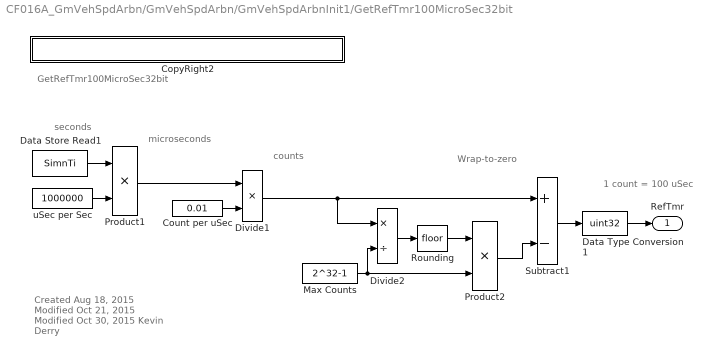
== system CF016A_GmVehSpdArbn/GmVehSpdArbn/GmVehSpdArbnInit1/GetRefTmr100MicroSec32bit ==
  note: 1 count = 100 uSec
  note: seconds
  note: microseconds
  note: counts
  note: Wrap-to-zero
  note: GetRefTmr100MicroSec32bit
  note: Created Aug 18, 2015
      | Modified Oct 21, 2015
      | Modified Oct 30, 2015
      | Kevin Derry
  CopyRight2 : Subsystem  Description=|  mask(Copyright Information){none=on}
      | Copyright info block.                                               
      |                                                                     
      | Place copyright information at the top of every subsystem in design.
      mask prompts: none "No parameters"
      mask help: Place copyright information at the top of every subsystem in design.
      mask Display:
      | NxtrConf = 'Nexteer Confidential';
      | 
      | sys = bdroot; %handle for the current model ("system")
      | first = get_param(sys,'Created');
      | if(isempty(first))
      |     first = datestr(now,'yyyy');
      | else
      |     first = first(end-3:end);  %year is last four digits
      | end
      | 
      | last = get_param(sys,'LastModifiedDate');
      | if isempty(last)
      |     last = datestr(now,'yyyy');
      | else
      |     last = last(end-3:end);
      | end
      | 
      | if strcmp(first,last)
      |     fprintf('%s -- Copyright %s Nexteer',NxtrConf,first)
      | else
      |     fprintf('%s -- %s%s- %s Nexteer',NxtrConf,char(169),first,last)
      | end
  Count per uSec : Constant  Value=0.01
  Data Store Read1 : DataStoreRead  DataStoreName=SimnTi
  Data Type Conversion1 : DataTypeConversion  OutDataTypeStr=uint32
  Divide1 : Product  Inputs=**
  Divide2 : Product  Inputs=*/
  Max Counts : Constant  Value=2^32-1
  Product1 : Product
  Product2 : Product
  Rounding : Rounding
  Subtract1 : Sum  Inputs=+-
  uSec per Sec : Constant  Value=1000000
  RefTmr : Outport
  wires:
  Product2/1 -> Subtract1/2
  Subtract1/1 -> Data Type Conversion1/1
  Rounding/1 -> Product2/1
  Divide2/1 -> Rounding/1
  Max Counts/1 -> Divide2/2, Product2/2
  Divide1/1 -> Divide2/1, Subtract1/1
  Product1/1 -> Divide1/1
  Count per uSec/1 -> Divide1/2
  uSec per Sec/1 -> Product1/2
  Data Type Conversion1/1 -> RefTmr/1
  Data Store Read1/1 -> Product1/1

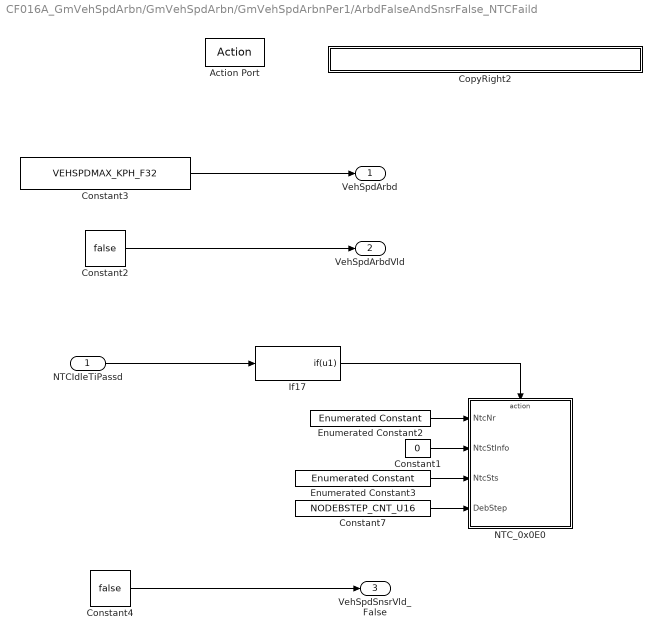
== system CF016A_GmVehSpdArbn/GmVehSpdArbn/GmVehSpdArbnPer1/ArbdFalseAndSnsrFalse_NTCFaild ==
  NTCIdleTiPassd : Inport  RequirementInfo="{'linktype_rmi_doors' '0000c6e6 (/GM T1XX/SubSystem Specifications/Customer Functions/CF016A GM Vehicle Speed Arbitration)' '#55' 'true' 'REQ:  55' '' } %GIDa_1cee0ec7_c7dd_4d16_bb3f_22ce6da4bd48"  OutDataTypeStr=boolean
  Action Port : ActionPort  ActionType=then
  Constant1 : Constant  RequirementInfo="{'linktype_rmi_doors' '0000c6e6 (/GM T1XX/SubSystem Specifications/Customer Functions/CF016A GM Vehicle Speed Arbitration)' '#55' 'true' 'REQ:  55' '' } %GIDa_38570a4d_8180_46ec_b175_4ff4536d7ca4"  Value=0
  Constant2 : Constant  RequirementInfo="{'linktype_rmi_doors' '0000c6e6 (/GM T1XX/SubSystem Specifications/Customer Functions/CF016A GM Vehicle Speed Arbitration)' '#201' 'true' 'REQ:  201' '' } %GIDa_da814d33_d5e2_43c9_97d3_6d420715544d"  Value=false  OutDataTypeStr=boolean
      settings: AttributesFormatString=%<OutDataTypeStr>
  Constant3 : Constant  RequirementInfo="{'linktype_rmi_doors' '0000c6e6 (/GM T1XX/SubSystem Specifications/Customer Functions/CF016A GM Vehicle Speed Arbitration)' '#201' 'true' 'REQ:  201' '' } %GIDa_b46124ad_ec86_4edb_90c0_b891f3c900cd"  Value=VEHSPDMAX_KPH_F32  OutDataTypeStr=single
      settings: AttributesFormatString=%<OutDataTypeStr>
  Constant4 : Constant  RequirementInfo="{'linktype_rmi_doors' '0000c6e6 (/GM T1XX/SubSystem Specifications/Customer Functions/CF016A GM Vehicle Speed Arbitration)' '#216' 'true' 'REQ:  216' '' } %GIDa_132db536_d186_47ff_b139_0bdfcec16fcb"  Value=false  OutDataTypeStr=boolean
      settings: AttributesFormatString=%<OutDataTypeStr>
  Constant7 : Constant  RequirementInfo="{'linktype_rmi_doors' '0000c6e6 (/GM T1XX/SubSystem Specifications/Customer Functions/CF016A GM Vehicle Speed Arbitration)' '#55' 'true' 'REQ:  55' '' } %GIDa_8e6884c7_a92c_4cf0_a40b_6de5e8b6e97f"  Value=NODEBSTEP_CNT_U16
  CopyRight2 : Subsystem  Description=|  mask(Copyright Information){none=on}
      | Copyright info block.                                               
      |                                                                     
      | Place copyright information at the top of every subsystem in design.
      mask prompts: none "No parameters"
      mask help: Place copyright information at the top of every subsystem in design.
      mask Display:
      | NxtrConf = 'Nexteer Confidential';
      | 
      | sys = bdroot; %handle for the current model ("system")
      | first = get_param(sys,'Created');
      | if(isempty(first))
      |     first = datestr(now,'yyyy');
      | else
      |     first = first(end-3:end);  %year is last four digits
      | end
      | 
      | last = get_param(sys,'LastModifiedDate');
      | if isempty(last)
      |     last = datestr(now,'yyyy');
      | else
      |     last = last(end-3:end);
      | end
      | 
      | if strcmp(first,last)
      |     fprintf('%s -- Copyright %s Nexteer',NxtrConf,first)
      | else
      |     fprintf('%s -- %s%s- %s Nexteer',NxtrConf,char(169),first,last)
      | end
  Enumerated Constant2 : simulink/Sources/Enumerated Constant  RequirementInfo="{'linktype_rmi_doors' '0000c6e6 (/GM T1XX/SubSystem Specifications/Customer Functions/CF016A GM Vehicle Speed Arbitration)' '#55' 'true' 'REQ:  55' '' } %GIDa_7367d177_40d0_4af4_b31b_4e45c9c7cab5"  OutDataTypeStr=Enum: NtcNr1  Value=NtcNr1.NTCNR_0X0E0  SampleTime=inf
  Enumerated Constant3 : simulink/Sources/Enumerated Constant  RequirementInfo="{'linktype_rmi_doors' '0000c6e6 (/GM T1XX/SubSystem Specifications/Customer Functions/CF016A GM Vehicle Speed Arbitration)' '#55' 'true' 'REQ:  55' '' } %GIDa_a858f8b7_33e3_47a8_8507_40965f315a45"  OutDataTypeStr=Enum: NtcSts1  Value=NtcSts1.NTCSTS_FAILD  SampleTime=inf
  If17 : If  RequirementInfo="{'linktype_rmi_doors' '0000c6e6 (/GM T1XX/SubSystem Specifications/Customer Functions/CF016A GM Vehicle Speed Arbitration)' '#55' 'true' 'REQ:  55' '' } %GIDa_95b1a695_556f_4bdf_82b2_bd99c1838ee0"  IfExpression=u1  ShowElse=off
      settings: AttributesFormatString=%<Priority>
  NTC_0x0E0 : Subsystem  RequirementInfo="{'linktype_rmi_doors' '0000c6e6 (/GM T1XX/SubSystem Specifications/Customer Functions/CF016A GM Vehicle Speed Arbitration)' '#55' 'true' 'REQ:  55' '' } %GIDa_d505394d_4557_497d_8832_7793d2bdfb5b"  mask(SetNTC){}
      mask help: SetNTC library block
  VehSpdArbd : Outport  RequirementInfo="{'linktype_rmi_doors' '0000c6e6 (/GM T1XX/SubSystem Specifications/Customer Functions/CF016A GM Vehicle Speed Arbitration)' '#201' 'true' 'REQ:  201' '' } %GIDa_c34adab8_c744_4205_8a49_9db71c9c59e2"
  VehSpdArbdVld : Outport  RequirementInfo="{'linktype_rmi_doors' '0000c6e6 (/GM T1XX/SubSystem Specifications/Customer Functions/CF016A GM Vehicle Speed Arbitration)' '#201' 'true' 'REQ:  201' '' } %GIDa_8a7a5b0a_f314_4f2b_83ec_e79d9bac700f"  Port=2
  VehSpdSnsrVld_False : Outport  RequirementInfo="{'linktype_rmi_doors' '0000c6e6 (/GM T1XX/SubSystem Specifications/Customer Functions/CF016A GM Vehicle Speed Arbitration)' '#216' 'true' 'REQ:  216' '' } %GIDa_8219bf46_2668_44cd_9756_c542298b020b"  Port=3
  wires:
  Constant3/1 -> VehSpdArbd/1
  Constant2/1 -> VehSpdArbdVld/1
  If17/1 -> NTC_0x0E0/Action
  Enumerated Constant3/1 -> NTC_0x0E0/3(NtcSts)
  Constant7/1 -> NTC_0x0E0/4(DebStep)
  Constant1/1 -> NTC_0x0E0/2(NtcStInfo)
  Enumerated Constant2/1 -> NTC_0x0E0/1(NtcNr)
  Constant4/1 -> VehSpdSnsrVld_False/1
  NTCIdleTiPassd/1 -> If17/1

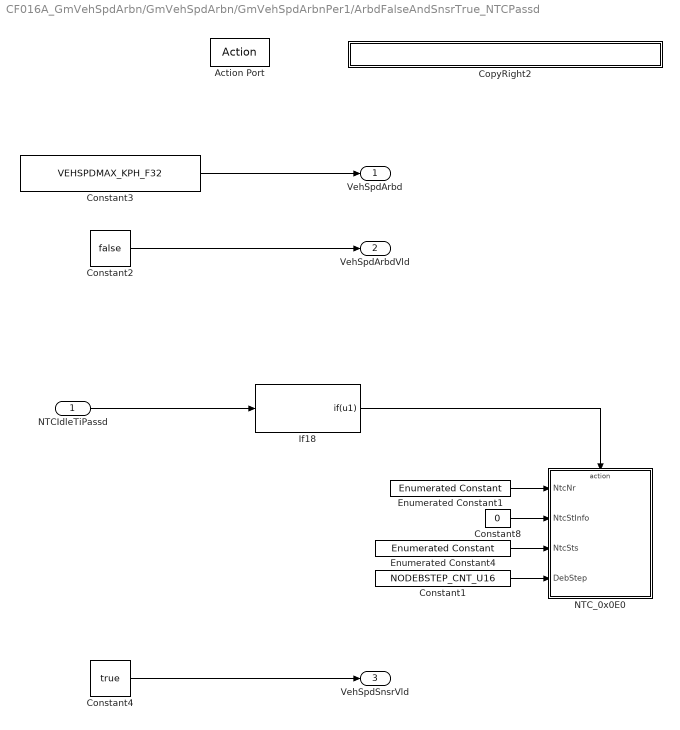
== system CF016A_GmVehSpdArbn/GmVehSpdArbn/GmVehSpdArbnPer1/ArbdFalseAndSnsrTrue_NTCPassd ==
  NTCIdleTiPassd : Inport  RequirementInfo="{'linktype_rmi_doors' '0000c6e6 (/GM T1XX/SubSystem Specifications/Customer Functions/CF016A GM Vehicle Speed Arbitration)' '#55' 'true' 'REQ:  55' '' } %GIDa_ea98937e_8d35_4b9d_92e7_fa2bf191a1f6"  OutDataTypeStr=boolean
  Action Port : ActionPort  ActionType=elseif
  Constant1 : Constant  RequirementInfo="{'linktype_rmi_doors' '0000c6e6 (/GM T1XX/SubSystem Specifications/Customer Functions/CF016A GM Vehicle Speed Arbitration)' '#55' 'true' 'REQ:  55' '' } %GIDa_48c90434_65d9_4695_bc5e_13689863c1e6"  Value=NODEBSTEP_CNT_U16
  Constant2 : Constant  RequirementInfo="{'linktype_rmi_doors' '0000c6e6 (/GM T1XX/SubSystem Specifications/Customer Functions/CF016A GM Vehicle Speed Arbitration)' '#201' 'true' 'REQ:  201' '' } %GIDa_7f2df84c_a00a_4ae7_8298_fb52d0c22ad7"  Value=false  OutDataTypeStr=boolean
      settings: AttributesFormatString=%<OutDataTypeStr>
  Constant3 : Constant  RequirementInfo="{'linktype_rmi_doors' '0000c6e6 (/GM T1XX/SubSystem Specifications/Customer Functions/CF016A GM Vehicle Speed Arbitration)' '#201' 'true' 'REQ:  201' '' } %GIDa_cfef0008_79bc_49ca_b258_3157e3d22f30"  Value=VEHSPDMAX_KPH_F32  OutDataTypeStr=single
      settings: AttributesFormatString=%<OutDataTypeStr>
  Constant4 : Constant  RequirementInfo="{'linktype_rmi_doors' '0000c6e6 (/GM T1XX/SubSystem Specifications/Customer Functions/CF016A GM Vehicle Speed Arbitration)' '#216' 'true' 'REQ:  216' '' } %GIDa_0ed9b788_538b_449e_8c4f_c22b3fbfaee9"  Value=true  OutDataTypeStr=boolean
      settings: AttributesFormatString=%<OutDataTypeStr>
  Constant8 : Constant  RequirementInfo="{'linktype_rmi_doors' '0000c6e6 (/GM T1XX/SubSystem Specifications/Customer Functions/CF016A GM Vehicle Speed Arbitration)' '#55' 'true' 'REQ:  55' '' } %GIDa_410cc41e_1718_4346_a63d_7d112e684ea3"  Value=0
  CopyRight2 : Subsystem  Description=|  mask(Copyright Information){none=on}
      | Copyright info block.                                               
      |                                                                     
      | Place copyright information at the top of every subsystem in design.
      mask prompts: none "No parameters"
      mask help: Place copyright information at the top of every subsystem in design.
      mask Display:
      | NxtrConf = 'Nexteer Confidential';
      | 
      | sys = bdroot; %handle for the current model ("system")
      | first = get_param(sys,'Created');
      | if(isempty(first))
      |     first = datestr(now,'yyyy');
      | else
      |     first = first(end-3:end);  %year is last four digits
      | end
      | 
      | last = get_param(sys,'LastModifiedDate');
      | if isempty(last)
      |     last = datestr(now,'yyyy');
      | else
      |     last = last(end-3:end);
      | end
      | 
      | if strcmp(first,last)
      |     fprintf('%s -- Copyright %s Nexteer',NxtrConf,first)
      | else
      |     fprintf('%s -- %s%s- %s Nexteer',NxtrConf,char(169),first,last)
      | end
  Enumerated Constant1 : simulink/Sources/Enumerated Constant  RequirementInfo="{'linktype_rmi_doors' '0000c6e6 (/GM T1XX/SubSystem Specifications/Customer Functions/CF016A GM Vehicle Speed Arbitration)' '#55' 'true' 'REQ:  55' '' } %GIDa_b219b4be_f5e6_4376_b10b_cd4b9d25b1b0"  OutDataTypeStr=Enum: NtcNr1  Value=NtcNr1.NTCNR_0X0E0  SampleTime=inf
  Enumerated Constant4 : simulink/Sources/Enumerated Constant  RequirementInfo="{'linktype_rmi_doors' '0000c6e6 (/GM T1XX/SubSystem Specifications/Customer Functions/CF016A GM Vehicle Speed Arbitration)' '#55' 'true' 'REQ:  55' '' } %GIDa_07ad565e_9b7f_464d_b0f3_60f534ebaf4b"  OutDataTypeStr=Enum: NtcSts1  Value=NtcSts1.NTCSTS_PASSD  SampleTime=inf
  If18 : If  RequirementInfo="{'linktype_rmi_doors' '0000c6e6 (/GM T1XX/SubSystem Specifications/Customer Functions/CF016A GM Vehicle Speed Arbitration)' '#55' 'true' 'REQ:  55' '' } %GIDa_febd9457_9624_49c5_b474_caa5da234fe0"  IfExpression=u1  ShowElse=off
      settings: AttributesFormatString=%<Priority>
  NTC_0x0E0 : Subsystem  RequirementInfo="{'linktype_rmi_doors' '0000c6e6 (/GM T1XX/SubSystem Specifications/Customer Functions/CF016A GM Vehicle Speed Arbitration)' '#55' 'true' 'REQ:  55' '' } %GIDa_325dcae8_63d7_4a36_b47a_3002bd5048ba"  mask(SetNTC){}
      mask help: SetNTC library block
  VehSpdArbd : Outport  RequirementInfo="{'linktype_rmi_doors' '0000c6e6 (/GM T1XX/SubSystem Specifications/Customer Functions/CF016A GM Vehicle Speed Arbitration)' '#201' 'true' 'REQ:  201' '' } %GIDa_5a2b06da_7da1_4c15_8e8a_e64399f2391e"
  VehSpdArbdVld : Outport  RequirementInfo="{'linktype_rmi_doors' '0000c6e6 (/GM T1XX/SubSystem Specifications/Customer Functions/CF016A GM Vehicle Speed Arbitration)' '#201' 'true' 'REQ:  201' '' } %GIDa_f0a23f13_69af_47b0_9d2a_c004505a54f6"  Port=2
  VehSpdSnsrVld : Outport  RequirementInfo="{'linktype_rmi_doors' '0000c6e6 (/GM T1XX/SubSystem Specifications/Customer Functions/CF016A GM Vehicle Speed Arbitration)' '#216' 'true' 'REQ:  216' '' } %GIDa_0a4a7de5_a034_4ced_ac3a_0fc8cb9c4640"  Port=3
  wires:
  Constant2/1 -> VehSpdArbdVld/1
  Constant3/1 -> VehSpdArbd/1
  If18/1 -> NTC_0x0E0/Action
  Enumerated Constant1/1 -> NTC_0x0E0/1(NtcNr)
  Enumerated Constant4/1 -> NTC_0x0E0/3(NtcSts)
  Constant1/1 -> NTC_0x0E0/4(DebStep)
  Constant8/1 -> NTC_0x0E0/2(NtcStInfo)
  Constant4/1 -> VehSpdSnsrVld/1
  NTCIdleTiPassd/1 -> If18/1

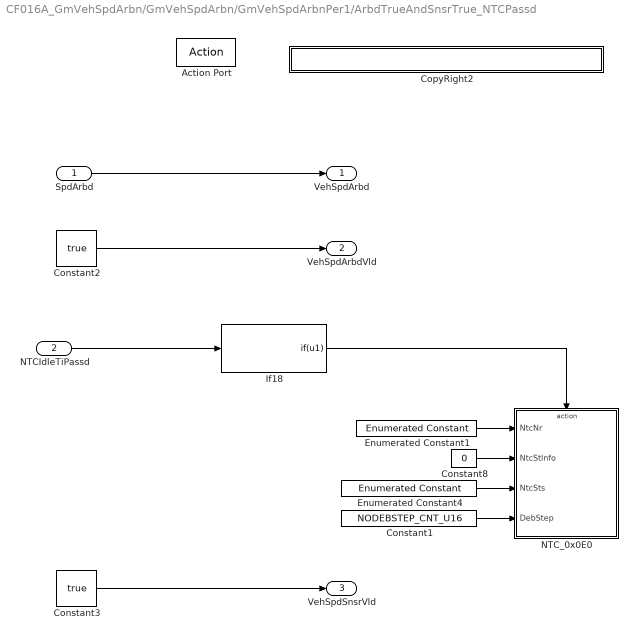
== system CF016A_GmVehSpdArbn/GmVehSpdArbn/GmVehSpdArbnPer1/ArbdTrueAndSnsrTrue_NTCPassd ==
  SpdArbd : Inport  RequirementInfo="{'linktype_rmi_doors' '0000c6e6 (/GM T1XX/SubSystem Specifications/Customer Functions/CF016A GM Vehicle Speed Arbitration)' '#201' 'true' 'REQ:  201' '' } %GIDa_2cd28403_f409_4b0d_a4ad_3f972e342b9c"
  NTCIdleTiPassd : Inport  RequirementInfo="{'linktype_rmi_doors' '0000c6e6 (/GM T1XX/SubSystem Specifications/Customer Functions/CF016A GM Vehicle Speed Arbitration)' '#55' 'true' 'REQ:  55' '' } %GIDa_1e41578b_7438_43d3_b9df_ab475a2050af"  Port=2  OutDataTypeStr=boolean
  Action Port : ActionPort  ActionType=else
  Constant1 : Constant  RequirementInfo="{'linktype_rmi_doors' '0000c6e6 (/GM T1XX/SubSystem Specifications/Customer Functions/CF016A GM Vehicle Speed Arbitration)' '#55' 'true' 'REQ:  55' '' } %GIDa_b38e3293_533d_4a72_9bd3_db93ba404680"  Value=NODEBSTEP_CNT_U16
  Constant2 : Constant  RequirementInfo="{'linktype_rmi_doors' '0000c6e6 (/GM T1XX/SubSystem Specifications/Customer Functions/CF016A GM Vehicle Speed Arbitration)' '#201' 'true' 'REQ:  201' '' } %GIDa_54cbd6ea_7017_4519_89a1_2b2ff899016e"  Value=true  OutDataTypeStr=boolean
      settings: AttributesFormatString=%<OutDataTypeStr>
  Constant3 : Constant  RequirementInfo="{'linktype_rmi_doors' '0000c6e6 (/GM T1XX/SubSystem Specifications/Customer Functions/CF016A GM Vehicle Speed Arbitration)' '#216' 'true' 'REQ:  216' '' } %GIDa_31b4124d_39fb_48f2_a229_d2538585466b"  Value=true  OutDataTypeStr=boolean
      settings: AttributesFormatString=%<OutDataTypeStr>
  Constant8 : Constant  RequirementInfo="{'linktype_rmi_doors' '0000c6e6 (/GM T1XX/SubSystem Specifications/Customer Functions/CF016A GM Vehicle Speed Arbitration)' '#55' 'true' 'REQ:  55' '' } %GIDa_98a683ad_0c8a_4c6e_8fcd_d982dd587fb3"  Value=0
  CopyRight2 : Subsystem  Description=|  mask(Copyright Information){none=on}
      | Copyright info block.                                               
      |                                                                     
      | Place copyright information at the top of every subsystem in design.
      mask prompts: none "No parameters"
      mask help: Place copyright information at the top of every subsystem in design.
      mask Display:
      | NxtrConf = 'Nexteer Confidential';
      | 
      | sys = bdroot; %handle for the current model ("system")
      | first = get_param(sys,'Created');
      | if(isempty(first))
      |     first = datestr(now,'yyyy');
      | else
      |     first = first(end-3:end);  %year is last four digits
      | end
      | 
      | last = get_param(sys,'LastModifiedDate');
      | if isempty(last)
      |     last = datestr(now,'yyyy');
      | else
      |     last = last(end-3:end);
      | end
      | 
      | if strcmp(first,last)
      |     fprintf('%s -- Copyright %s Nexteer',NxtrConf,first)
      | else
      |     fprintf('%s -- %s%s- %s Nexteer',NxtrConf,char(169),first,last)
      | end
  Enumerated Constant1 : simulink/Sources/Enumerated Constant  RequirementInfo="{'linktype_rmi_doors' '0000c6e6 (/GM T1XX/SubSystem Specifications/Customer Functions/CF016A GM Vehicle Speed Arbitration)' '#55' 'true' 'REQ:  55' '' } %GIDa_430dd0b6_63d2_4424_a17c_fb826818d427"  OutDataTypeStr=Enum: NtcNr1  Value=NtcNr1.NTCNR_0X0E0  SampleTime=inf
  Enumerated Constant4 : simulink/Sources/Enumerated Constant  RequirementInfo="{'linktype_rmi_doors' '0000c6e6 (/GM T1XX/SubSystem Specifications/Customer Functions/CF016A GM Vehicle Speed Arbitration)' '#55' 'true' 'REQ:  55' '' } %GIDa_3e72926b_2bc1_477e_b43a_0dde04cc7eb1"  OutDataTypeStr=Enum: NtcSts1  Value=NtcSts1.NTCSTS_PASSD  SampleTime=inf
  If18 : If  RequirementInfo="{'linktype_rmi_doors' '0000c6e6 (/GM T1XX/SubSystem Specifications/Customer Functions/CF016A GM Vehicle Speed Arbitration)' '#55' 'true' 'REQ:  55' '' } %GIDa_8c6b0a7e_b710_4d2f_9c86_be79d5a6a8b4"  IfExpression=u1  ShowElse=off
      settings: AttributesFormatString=%<Priority>
  NTC_0x0E0 : Subsystem  RequirementInfo="{'linktype_rmi_doors' '0000c6e6 (/GM T1XX/SubSystem Specifications/Customer Functions/CF016A GM Vehicle Speed Arbitration)' '#55' 'true' 'REQ:  55' '' } %GIDa_50e43290_1cf4_48bf_9db4_0d4ad04765ec"  mask(SetNTC){}
      mask help: SetNTC library block
  VehSpdArbd : Outport  RequirementInfo="{'linktype_rmi_doors' '0000c6e6 (/GM T1XX/SubSystem Specifications/Customer Functions/CF016A GM Vehicle Speed Arbitration)' '#201' 'true' 'REQ:  201' '' } %GIDa_76fb5f45_9bbc_4e67_b023_2f926d3f8c57"
  VehSpdArbdVld : Outport  RequirementInfo="{'linktype_rmi_doors' '0000c6e6 (/GM T1XX/SubSystem Specifications/Customer Functions/CF016A GM Vehicle Speed Arbitration)' '#201' 'true' 'REQ:  201' '' } %GIDa_0fd5aee5_09ea_43a7_8ad7_0cfaee6c0d61"  Port=2
  VehSpdSnsrVld : Outport  RequirementInfo="{'linktype_rmi_doors' '0000c6e6 (/GM T1XX/SubSystem Specifications/Customer Functions/CF016A GM Vehicle Speed Arbitration)' '#216' 'true' 'REQ:  216' '' } %GIDa_18066f3c_fbaa_4d3f_883a_52897e3515a6"  Port=3
  wires:
  Constant2/1 -> VehSpdArbdVld/1
  SpdArbd/1 -> VehSpdArbd/1
  If18/1 -> NTC_0x0E0/Action
  Enumerated Constant1/1 -> NTC_0x0E0/1(NtcNr)
  Enumerated Constant4/1 -> NTC_0x0E0/3(NtcSts)
  Constant1/1 -> NTC_0x0E0/4(DebStep)
  Constant8/1 -> NTC_0x0E0/2(NtcStInfo)
  Constant3/1 -> VehSpdSnsrVld/1
  NTCIdleTiPassd/1 -> If18/1
